simulink subsystem "PvtSubSys_PLAN_AP"  (R2020b)
settings: Solver=VariableStepAuto  StartTime=0.0  StopTime=10.0  RelTol=1e-3
undefined symbols (not defined in the file or in its folder): C_LongCtrl_0_Single, C_LongCtrl_0_Uint8, C_LongCtrl_Mph2Kph, magnitude, P_LongCtrl_accelTargAbsThrd, P_LongCtrl_AddVelAccelChange, P_LongCtrl_AddVelAccelThrd, P_LongCtrl_AddVelDistDesThrd, P_LongCtrl_AddVelEnable, P_LongCtrl_AddVelRefMsThrd, P_LongCtrl_ALaLowerChar, P_LongCtrl_ALaUpperCharEco, P_LongCtrl_ALaUpperCharNormal, P_LongCtrl_ALaUpperCharSport, P_LongCtrl_ALCAccLimitByDangerXAxis, P_LongCtrl_ALCAccLimitByDangerYAxis, P_LongCtrl_ALvAcceleLowerChar, P_LongCtrl_ALvAcceleUpperCharEco, P_LongCtrl_ALvAcceleUpperCharNormal, P_LongCtrl_ALvAcceleUpperCharSport, P_LongCtrl_CCaccelCCNeg2PosJerk, P_LongCtrl_CCaccelCCPosJerk, P_LongCtrl_CCaccelLowerIsLaneChange, P_LongCtrl_CCaccelMaxLCActive, P_LongCtrl_CCaccelMinECOAL, P_LongCtrl_CCaccelMinFastDecel, P_LongCtrl_CCaccelMinNoFastDecel, P_LongCtrl_CCaccelMinNormAL, P_LongCtrl_CCaccelMinSportAL, P_LongCtrl_CCaccelUpperCC, P_LongCtrl_CCaccelUpperCCSafeStop, P_LongCtrl_CCaMinNegAcceleLowerBand, P_LongCtrl_CCaMinNegAcceleUpperBand, P_LongCtrl_CCaMinPosAcceleLowerBand, P_LongCtrl_CCaMinPosAcceleUpperBand, P_LongCtrl_CCbECO, P_LongCtrl_CCbNorm, P_LongCtrl_CCbSport, P_LongCtrl_CCcoefESPSpd2IPSpd1, P_LongCtrl_CCcoefESPSpd2IPSpd2, P_LongCtrl_CCdecelCCJerk, P_LongCtrl_CCdecelCCJerkNegVLCInternalAcc, P_LongCtrl_CCfacNegAcceleLowerBand, P_LongCtrl_CCfacNegAcceleUpperBand, P_LongCtrl_CCfacPosAcceleLowerBand, P_LongCtrl_CCfacPosAcceleUpperBand, P_LongCtrl_CCkECO, P_LongCtrl_CCkNorm, P_LongCtrl_CCkSport, P_LongCtrl_CCLCIncSetSpdAdd, P_LongCtrl_CCLCIncSetSpdAddCntStartValue, P_LongCtrl_CCResumeDelayDeltaVel, P_LongCtrl_CCtAcceleTimeNeg, P_LongCtrl_CCtAcceleTimeNegCorrXAxis, P_LongCtrl_CCtAcceleTimeNegCorrYAxis, P_LongCtrl_CCtAcceleTimePos, P_LongCtrl_CCtAcceleTimePosCorrXAxis, P_LongCtrl_CCtAcceleTimePosCorrYAxis, P_LongCtrl_CCtStepVelPlan, P_LongCtrl_CCtTotVelPlan ... (+150)
libraries: simulink x62, TrueDurationTime x1
(part 5 of 7)

== system PvtSubSys_PLAN_AP/AP/AP/IC/CurvatureOfMapCalc/Chart/velSubjLimChar ==
  LongCtrl_IC_EHRV2_CurMatrixLP : Inport  OutDataTypeStr=single  PortDimensions=[1 10]
  f : TriggerPort  TriggerType=function-call  VariantControl=(inherit)
      settings: CopyFcn=Stateflow.SLINSF.SimulinkMan.removeBlockPreDeleteFcn  PreDeleteFcn=Stateflow.SLINSF.SimulinkMan.unsafePredeleteFcn
  1-D Lookup Table2 : Lookup_n-D  NumberOfTableDimensions=1  BreakpointsForDimension1=P_LongCtrl_ICCurvatureMapLimitSpdXAxis  Table=P_LongCtrl_ICCurvatureMapLimitSpdYAxis  ExtrapMethod=Clip  InternalRulePriority=Speed  RndMeth=Simplest  InputSameDT=on
  Gain2 : Gain  Gain=1/3.6
  velSubjLimMap : Outport
  wires:
  LongCtrl_IC_EHRV2_CurMatrixLP/1 -> 1-D Lookup Table2/1
  1-D Lookup Table2/1 -> Gain2/1
  Gain2/1 -> velSubjLimMap/1

== system PvtSubSys_PLAN_AP/AP/AP/IC/CurvatureOfMapCalc/LP ==
  LongCtrl_IC_EHRV2_CurMatrix : Inport  OutDataTypeStr=single  Partition=on  PartitionDimension=1  PartitionWidth=1  PartitionOffset=0
  Abs : Abs
  Abs1 : Abs
  Add : Sum  Inputs=--+  OutDataTypeStr=single
  Add5 : Sum  Inputs=+-
  Add6 : Sum
  Compare To Constant : simulink/Logic and Bit Operations/Compare To Constant  relop=>=  const=0.15  OutDataTypeStr=boolean
  Constant : Constant  Value=0  OutDataTypeStr=single
  Constant1 : Constant  Value=0.1  OutDataTypeStr=single
  Constant12 : Constant  Value=0.02  OutDataTypeStr=single
  For Each : ForEach  DisableCoverage=on
  Max : MinMax  Function=max
  Min : MinMax
  Product7 : Product  Inputs=*/
  Product8 : Product
  Sum of Elements2 : Sum  Inputs=+
  Switch : Switch  Criteria=u2 > Threshold
  Tapped Delay2 : simulink/Discrete/Tapped Delay  vinit=0.0  samptime=-1  NumDelays=3  DelayOrder=Oldest  includeCurrent=off
  Unit Delay : UnitDelay  SampleTime=-1  HasFrameUpgradeWarning=on
  LongCtrl_IC_EHRV2_CurMatrixLP : Outport  ConcatenationDimension=1
  wires:
  Unit Delay/1 -> Add6/2, Add5/2
  Constant1/1 -> Product7/2
  Min/1 -> Add/2
  Max/1 -> Add/1
  Sum of Elements2/1 -> Add/3
  Constant12/1 -> Product7/1
  Product7/1 -> Product8/1
  Add/1 -> Add5/1
  Add5/1 -> Product8/2
  Product8/1 -> Add6/1
  Add6/1 -> Switch/3
  Tapped Delay2/1 -> Sum of Elements2/1, Max/1, Min/1
  Abs/1 -> LongCtrl_IC_EHRV2_CurMatrixLP/1
  Abs1/1 -> Compare To Constant/1
  Compare To Constant/1 -> Switch/2
  LongCtrl_IC_EHRV2_CurMatrix/1 -> Abs1/1, Tapped Delay2/1
  Switch/1 -> Unit Delay/1, Abs/1
  Constant/1 -> Switch/1

== system PvtSubSys_PLAN_AP/AP/AP/IC/CurvatureOfRoadCalc/If Action Subsystem ==
  L1dC2V : Inport
  L1dC3V : Inport  Port=2
  R1dC2V : Inport  Port=3
  R1dC3V : Inport  Port=4
  L1dDisFront : Inport  Port=5
  R1dDisFront : Inport  Port=6
  L1bIsLineExist : Inport  Port=7
  R1bIsLineExis : Inport  Port=8
  velSubj : Inport  Port=9
  LongCtrl_Line_std : Inport  Port=10
  Action Port : ActionPort
  Abs : Abs
  Constant : Constant  Value=0  OutDataTypeStr=single
  Constant1 : Constant  Value=0  OutDataTypeStr=single
  CurvatureMix : Subsystem
  For Each Subsystem : Subsystem  TreatAsAtomicUnit=on
  Vector Concatenate : Concatenate
  Vector Concatenate1 : Concatenate
  Curvature : Outport
  wires:
  Vector Concatenate1/1 -> For Each Subsystem/4(R1dC3V)
  Constant1/1 -> Vector Concatenate1/1
  Constant/1 -> Vector Concatenate/1
  Vector Concatenate/1 -> For Each Subsystem/2(L1dC3V)
  Abs/1 -> CurvatureMix/1(In1)
  CurvatureMix/1(Out1) -> Curvature/1
  For Each Subsystem/1(Curvature) -> Abs/1  "Curvature"
  velSubj/1 -> For Each Subsystem/9(velSubj)  "velSubj"
  L1dC2V/1 -> For Each Subsystem/1(L1dC2V)
  R1dC2V/1 -> For Each Subsystem/3(R1dC2V)
  L1bIsLineExist/1 -> For Each Subsystem/7(L1bIsLineExist)
  R1bIsLineExis/1 -> For Each Subsystem/8(R1bIsLineExis)
  L1dC3V/1 -> Vector Concatenate/2
  L1dDisFront/1 -> For Each Subsystem/5(L1dDisFront)
  R1dDisFront/1 -> For Each Subsystem/6(R1dDisFront)
  R1dC3V/1 -> Vector Concatenate1/2
  LongCtrl_Line_std/1 -> CurvatureMix/2(LongCtrl_Line_std)

== system PvtSubSys_PLAN_AP/AP/AP/IC/CurvatureOfRoadCalc/If Action Subsystem1 ==
  Action Port : ActionPort
  Constant17 : Constant  Value=0  OutDataTypeStr=single
  Curvature : Outport
  wires:
  Constant17/1 -> Curvature/1

== system PvtSubSys_PLAN_AP/AP/AP/IC/CurvatureOfRoadCalc/LP2 ==
  In1 : Inport
  Add5 : Sum  Inputs=+-
  Add6 : Sum
  Constant12 : Constant  Value=0.02  OutDataTypeStr=single
  Constant13 : Constant  Value=0.3  OutDataTypeStr=single
  Product7 : Product  Inputs=*/
  Product8 : Product
  Unit Delay : UnitDelay  SampleTime=-1  HasFrameUpgradeWarning=on
  Out1 : Outport
  wires:
  Constant12/1 -> Product7/1
  Constant13/1 -> Product7/2
  Product7/1 -> Product8/1
  In1/1 -> Add5/1
  Product8/1 -> Add6/1
  Add6/1 -> Out1/1, Unit Delay/1
  Unit Delay/1 -> Add5/2, Add6/2
  Add5/1 -> Product8/2

== system PvtSubSys_PLAN_AP/AP/AP/IC/Subsystem1/Subsystem ==
  In1 : Inport
  Add : Sum  Inputs=--+  OutDataTypeStr=single
  Add1 : Sum  Inputs=--+  OutDataTypeStr=single
  Demux : Demux  Outputs=2
  Max : MinMax  Function=max
  Max1 : MinMax  Function=max
  Min : MinMax
  Min1 : MinMax
  Mux : Mux  Inputs=2
  Sum of Elements1 : Sum  Inputs=+
  Sum of Elements2 : Sum  Inputs=+
  Tapped Delay1 : simulink/Discrete/Tapped Delay  vinit=0.0  samptime=-1  NumDelays=3  DelayOrder=Oldest  includeCurrent=off
  Tapped Delay2 : simulink/Discrete/Tapped Delay  vinit=0.0  samptime=-1  NumDelays=3  DelayOrder=Oldest  includeCurrent=off
  Line_stdK1 : Outport
  wires:
  Tapped Delay2/1 -> Max/1, Min/1, Sum of Elements2/1
  Max/1 -> Add/1
  Min/1 -> Add/2
  Sum of Elements2/1 -> Add/3
  In1/1 -> Demux/1
  Sum of Elements1/1 -> Add1/3
  Min1/1 -> Add1/2
  Max1/1 -> Add1/1
  Tapped Delay1/1 -> Sum of Elements1/1, Min1/1, Max1/1
  Demux/1 -> Tapped Delay1/1
  Demux/2 -> Tapped Delay2/1
  Add1/1 -> Mux/1
  Add/1 -> Mux/2
  Mux/1 -> Line_stdK1/1

== system PvtSubSys_PLAN_AP/AP/AP/IC/Subsystem1/Subsystem1 ==
  In1 : Inport
  Demux4 : Demux  Outputs=2
  Gain : Gain  Gain=0.04  OutDataTypeStr=single
  Gain1 : Gain  Gain=0.04  ParamDataTypeStr=single
  Mux1 : Mux  Inputs=2
  Sum of Elements : Sum  Inputs=+
  Sum of Elements1 : Sum  Inputs=+
  Tapped Delay : simulink/Discrete/Tapped Delay  vinit=0.0  samptime=-1  NumDelays=25  DelayOrder=Oldest  includeCurrent=off
  Tapped Delay1 : simulink/Discrete/Tapped Delay  vinit=0.0  samptime=-1  NumDelays=25  DelayOrder=Oldest  includeCurrent=off
  Out1 : Outport
  wires:
  Sum of Elements1/1 -> Gain1/1
  Mux1/1 -> Out1/1
  Gain1/1 -> Mux1/2
  Tapped Delay/1 -> Sum of Elements/1
  Demux4/1 -> Tapped Delay/1
  Sum of Elements/1 -> Gain/1
  Gain/1 -> Mux1/1
  Tapped Delay1/1 -> Sum of Elements1/1
  Demux4/2 -> Tapped Delay1/1
  In1/1 -> Demux4/1

== system PvtSubSys_PLAN_AP/AP/AP/SJ/DeceleToStop/DeceleToStop/DresCalc ==
  distTargRel : Inport  OutDataTypeStr=single  PortDimensions=1
  f : TriggerPort  TriggerType=function-call  VariantControl=Variant
      settings: CopyFcn=Stateflow.SLINSF.SimulinkMan.removeBlockPreDeleteFcn  PreDeleteFcn=Stateflow.SLINSF.SimulinkMan.unsafePredeleteFcn
  Add : Sum  Inputs=+-
  P_LongCtrl_SJdStop : Constant  Value=P_LongCtrl_SJdStop
  distRes : Outport
  wires:
  P_LongCtrl_SJdStop/1 -> Add/2
  Add/1 -> distRes/1  "distRes"
  distTargRel/1 -> Add/1  "distTargRel"

== system PvtSubSys_PLAN_AP/AP/AP/SJ/DeceleToStop/DeceleToStop/VxTargetCalc ==
  velSubj : Inport  OutDataTypeStr=single  PortDimensions=1
  velTargetRel : Inport  Port=2  OutDataTypeStr=single  PortDimensions=1
  f : TriggerPort  TriggerType=function-call  VariantControl=Variant
      settings: CopyFcn=Stateflow.SLINSF.SimulinkMan.removeBlockPreDeleteFcn  PreDeleteFcn=Stateflow.SLINSF.SimulinkMan.unsafePredeleteFcn
  Add : Sum
  velTargetAbs : Outport
  wires:
  Add/1 -> velTargetAbs/1  "velTargetAbs"
  velSubj/1 -> Add/1  "velSubj"
  velTargetRel/1 -> Add/2  "velTargetRel"

== system PvtSubSys_PLAN_AP/AP/AP/SJ/DisBar/ACC_DisplayBar1 ==
  TimeGap : Inport
  DesireDistance : Inport  Port=2
  ACCmode : Inport  Port=3
  TargetRange : Inport  Port=4  Partition=on  PartitionDimension=1  PartitionWidth=1  PartitionOffset=0
  Scale : Inport  Port=5
  TargetExist : Inport  Port=6  Partition=on  PartitionDimension=1  PartitionWidth=1  PartitionOffset=0
  ACC_DisplayBar : MATLAB Function  TreatAsAtomicUnit=on
  For Each : ForEach  DisableCoverage=on
  Unit Delay34 : UnitDelay  SampleTime=-1  HasFrameUpgradeWarning=on
  Signal_ACC_TgtObjBarDisp : Outport  ConcatenationDimension=1
  wires:
  TargetExist/1 -> ACC_DisplayBar/6(TargetExist)  "TargetExist"
  Scale/1 -> ACC_DisplayBar/5(Scale)  "Scale"
  TargetRange/1 -> ACC_DisplayBar/4(TargetRange)  "TargetRange"
  ACCmode/1 -> ACC_DisplayBar/3(ACCmode)  "ACCmode"
  DesireDistance/1 -> ACC_DisplayBar/2(DesireDistance)  "DesireDistance"
  TimeGap/1 -> ACC_DisplayBar/1(TimeGap)  "TimeGap"
  Unit Delay34/1 -> ACC_DisplayBar/7(DisplayBarK1)
  ACC_DisplayBar/1(DisplayBar) -> Unit Delay34/1, Signal_ACC_TgtObjBarDisp/1  "Signal_ACC_TgtObjBarDisp"

== system PvtSubSys_PLAN_AP/AP/AP/SJ/TakeOver/Gap ==
  distTargetRel : Inport
  velSubj : Inport  Port=2
  Constant : Constant  Value=0.1  OutDataTypeStr=single
  MinMax : MinMax  Function=max  Inputs=2
  Product : Product  Inputs=*/
  gap : Outport
  wires:
  MinMax/1 -> Product/2
  Constant/1 -> MinMax/2
  Product/1 -> gap/1
  velSubj/1 -> MinMax/1
  distTargetRel/1 -> Product/1

== system PvtSubSys_PLAN_AP/AP/AP/FollowCtrl/DecelToStopCtrl/DecelToStopCtrl/P_LongCtrl_velSubjThresEnableStopAdd ==
  distTargRel : Inport
  velSubjThresForceStop : Inport  Port=2
  1-D Lookup Table : Lookup_n-D  NumberOfTableDimensions=1  BreakpointsForDimension1=P_LongCtrl_FollowvelSubjThresEnableStopAddXAxis  Table=P_LongCtrl_FollowvelSubjThresEnableStopAddYAxis  ExtrapMethod=Clip  InternalRulePriority=Speed  RndMeth=Simplest  InputSameDT=on
  1-D Lookup Table1 : Lookup_n-D  NumberOfTableDimensions=1  BreakpointsForDimension1=P_LongCtrl_FollowaccelFollowDesThresEnableStopXAxis  Table=P_LongCtrl_FollowaccelFollowDesThresEnableStopYAxis  ExtrapMethod=Clip  InternalRulePriority=Speed  RndMeth=Simplest  InputSameDT=on
  Add : Sum  Inputs=+-
  Add1 : Sum
  Constant : Constant  Value=P_LongCtrl_FollowDistDiff2VelSubjThresEnableStop
  Lookup Table Dynamic : simulink/Lookup Tables/Lookup Table Dynamic  LookUpMeth=Interpolation-Use End Values  OutDataType=fixdt('single')  OutScaling=[]  OutputDataTypeScalingMode=Specify via dialog  OutDataTypeStr=single  DoSatur=off
  P_LongCtrl_FollowdistDesStopMin : Constant  Value=P_LongCtrl_FollowdistDesStopMin  OutDataTypeStr=single
  P_LongCtrl_FollowvelSubjThresEnableStop : Constant  Value=P_LongCtrl_FollowvelSubjThresEnableStop  OutDataTypeStr=single
  P_LongCtrl_FollowvelSubjThresEnableStop1 : Constant  Value=P_LongCtrl_FollowVelSubjForceStopEnable  OutDataTypeStr=single
  Switch : Switch  Criteria=u2 > Threshold
  Vector Concatenate : Concatenate
  accelFollowDesThresEnableStop : Outport
  velSubjThresEnableStopAdd : Outport  Port=2
  velSubjThresForceStopStationaryTarget : Outport  Port=3
  wires:
  distTargRel/1 -> 1-D Lookup Table1/1, Add/2
  P_LongCtrl_FollowdistDesStopMin/1 -> Add/1
  Add/1 -> Lookup Table Dynamic/1, 1-D Lookup Table/1
  1-D Lookup Table/1 -> Add1/2, velSubjThresEnableStopAdd/1  "LongCtrl_velSubjThresEnableStopAdd"
  1-D Lookup Table1/1 -> accelFollowDesThresEnableStop/1  "LongCtrl_accelFollowDesThresEnableStop"
  Constant/1 -> Lookup Table Dynamic/2
  velSubjThresForceStop/1 -> Vector Concatenate/1
  Add1/1 -> Switch/3, Vector Concatenate/2
  Vector Concatenate/1 -> Lookup Table Dynamic/3
  Switch/1 -> velSubjThresForceStopStationaryTarget/1  "LongCtrl_velSubjThresForceStopStationaryTarget"
  P_LongCtrl_FollowvelSubjThresEnableStop/1 -> Add1/1
  P_LongCtrl_FollowvelSubjThresEnableStop1/1 -> Switch/2
  Lookup Table Dynamic/1 -> Switch/1

== system PvtSubSys_PLAN_AP/AP/AP/FollowCtrl/DecelToStopCtrl/DecelToStopCtrl/Subsystem ==
  axvRoadSlopeMs2 : Inport
  P_LongCtrl_FollowaccelForceStopMinChar : Lookup_n-D  NumberOfTableDimensions=1  BreakpointsForDimension1=P_LongCtrl_FollowaccelForceStopMinCharXAxis  Table=P_LongCtrl_FollowaccelForceStopMinCharYAxis  ExtrapMethod=Clip  InternalRulePriority=Speed  OutDataTypeStr=single  RndMeth=Simplest  InputSameDT=on
  P_LongCtrl_jerkForceStopChar : Lookup_n-D  NumberOfTableDimensions=1  BreakpointsForDimension1=P_LongCtrl_FollowjerkForceStopCharXAxis  Table=P_LongCtrl_FollowjerkForceStopCharYAxis  ExtrapMethod=Clip  InternalRulePriority=Speed  RndMeth=Simplest  InputSameDT=on
  P_LongCtrl_velSubjThresForceStopChar : Lookup_n-D  NumberOfTableDimensions=1  BreakpointsForDimension1=P_LongCtrl_FollowVelSubjThresForceStopXAxis  Table=P_LongCtrl_FollowVelSubjThresForceStopYAxis  ExtrapMethod=Clip  InternalRulePriority=Speed  RndMeth=Simplest  InputSameDT=on
  velSubjThresForceStop : Outport
  jerkForceStop : Outport  Port=2
  accelForceMin : Outport  Port=3
  wires:
  axvRoadSlopeMs2/1 -> P_LongCtrl_FollowaccelForceStopMinChar/1, P_LongCtrl_jerkForceStopChar/1, P_LongCtrl_velSubjThresForceStopChar/1
  P_LongCtrl_velSubjThresForceStopChar/1 -> velSubjThresForceStop/1  "LongCtrl_velSubjThresForceStop"
  P_LongCtrl_jerkForceStopChar/1 -> jerkForceStop/1  "LongCtrl_jerkForceStop"
  P_LongCtrl_FollowaccelForceStopMinChar/1 -> accelForceMin/1  "LongCtrl_accelForceMin"

== system PvtSubSys_PLAN_AP/AP/AP/FollowCtrl/FollowBandJerkCalc/DecelFollowJerkCalc/OverrideJerk/lowerJerkOverrideCalc ==
  VlcInternalAccK1 : Inport  OutDataTypeStr=single  PortDimensions=1
  f : TriggerPort  TriggerType=function-call  VariantControl=Variant
      settings: CopyFcn=Stateflow.SLINSF.SimulinkMan.removeBlockPreDeleteFcn  PreDeleteFcn=Stateflow.SLINSF.SimulinkMan.unsafePredeleteFcn
  1-D Lookup Table : Lookup_n-D  NumberOfTableDimensions=1  BreakpointsForDimension1=[0 1 2 3]  Table=[-4 -10 -20 -30]  ExtrapMethod=Clip  InternalRulePriority=Speed  RndMeth=Simplest  InputSameDT=on
  lowerJerkOverride : Outport
  wires:
  1-D Lookup Table/1 -> lowerJerkOverride/1
  VlcInternalAccK1/1 -> 1-D Lookup Table/1

== system PvtSubSys_PLAN_AP/AP/AP/IC/CurvatureOfRoadCalc/If Action Subsystem/CurvatureMix ==
  In1 : Inport
  LongCtrl_Line_std : Inport  Port=2
  2-D Lookup Table1 : Lookup_n-D  BreakpointsForDimension1=P_LongCtrl_ICcoefCurvatureCharX1  BreakpointsForDimension2=P_LongCtrl_ICcoefCurvatureCharX2  Table=P_LongCtrl_ICcoefCurvatureCharY  ExtrapMethod=Clip  InternalRulePriority=Speed  RndMeth=Simplest  InputSameDT=on
      settings: InputPortMap=u0,u1
  Add : Sum  Inputs=+-
  Add1 : Sum
  Constant : Constant  OutDataTypeStr=single
  Demux : Demux  Outputs=2
  LP : Subsystem
  Product : Product
  Product1 : Product
  Signal Conversion : SignalConversion  OverrideOpt=off
  Signal Conversion1 : SignalConversion  OverrideOpt=off
  Out1 : Outport
  wires:
  Signal Conversion1/1 -> Product1/2, 2-D Lookup Table1/2  "LongCtrl_curvatureWithC3"
  Signal Conversion/1 -> Product/1, 2-D Lookup Table1/1  "LongCtrl_curvatureNoC3"
  Demux/1 -> Signal Conversion/1
  Add1/1 -> LP/1(In1)  "LongCtrl_curvatureForCurveDecelRaw"
  Demux/2 -> Signal Conversion1/1
  In1/1 -> Demux/1
  2-D Lookup Table1/1 -> Product/2, Add/2  "LongCtrl_coefCurvatureNoC3"
  Product1/1 -> Add1/2
  Product/1 -> Add1/1
  Add/1 -> Product1/1  "LongCtrl_coefCurvatureWithC3"
  Constant/1 -> Add/1
  LP/1(Out1) -> Out1/1
  LongCtrl_Line_std/1 -> LP/2(LongCtrl_Line_std)

== system PvtSubSys_PLAN_AP/AP/AP/IC/CurvatureOfRoadCalc/If Action Subsystem/For Each Subsystem ==
  L1dC2V : Inport
  L1dC3V : Inport  Port=2  Partition=on  PartitionDimension=1  PartitionWidth=1  PartitionOffset=0
  R1dC2V : Inport  Port=3
  R1dC3V : Inport  Port=4  Partition=on  PartitionDimension=1  PartitionWidth=1  PartitionOffset=0
  L1dDisFront : Inport  Port=5
  R1dDisFront : Inport  Port=6
  L1bIsLineExist : Inport  Port=7
  R1bIsLineExis : Inport  Port=8
  velSubj : Inport  Port=9
  CurvatureChar : Stateflow chart  TreatAsAtomicUnit=on
  For Each : ForEach  DisableCoverage=on
  Curvature : Outport  ConcatenationDimension=1
  wires:
  CurvatureChar/1(CurvatureIFC) -> Curvature/1  "Curvature"
  R1dC3V/1 -> CurvatureChar/7(GetR1dC3V)
  R1bIsLineExis/1 -> CurvatureChar/2(R1bIsLineExis)
  L1dDisFront/1 -> CurvatureChar/5(GetL1dDisFront)
  L1dC3V/1 -> CurvatureChar/4(GetL1dC3V)
  L1bIsLineExist/1 -> CurvatureChar/1(L1bIsLineExist)
  L1dC2V/1 -> CurvatureChar/3(GetL1dC2V)
  R1dC2V/1 -> CurvatureChar/6(GetR1dC2V)
  R1dDisFront/1 -> CurvatureChar/8(GetR1dDisFront)
  velSubj/1 -> CurvatureChar/9(velSubj)  "velSubj"

== system PvtSubSys_PLAN_AP/AP/AP/IC/CurvatureOfRoadCalc/If Action Subsystem/CurvatureMix/LP ==
  In1 : Inport
  LongCtrl_Line_std : Inport  Port=2
  1-D Lookup Table : Lookup_n-D  NumberOfTableDimensions=1  BreakpointsForDimension1=[0 0.3 0.6 0.9 1.2 1.5]  Table=[0.3 0.3 0.6 0.9 1.2 1.5]  InternalRulePriority=Speed  RndMeth=Simplest  InputSameDT=on
  Add : Sum  Inputs=--+  OutDataTypeStr=single
  Add5 : Sum  Inputs=+-
  Add6 : Sum
  Constant12 : Constant  Value=0.02  OutDataTypeStr=single
  Max : MinMax  Function=max
  Min : MinMax
  Product7 : Product  Inputs=*/
  Product8 : Product
  Sum of Elements2 : Sum  Inputs=+
  Tapped Delay2 : simulink/Discrete/Tapped Delay  vinit=0.0  samptime=-1  NumDelays=3  DelayOrder=Oldest  includeCurrent=off
  Unit Delay : UnitDelay  SampleTime=-1  HasFrameUpgradeWarning=on
  Out1 : Outport
  wires:
  Add5/1 -> Product8/2
  Unit Delay/1 -> Add6/2, Add5/2
  Add6/1 -> Unit Delay/1, Out1/1
  Product8/1 -> Add6/1
  Add/1 -> Add5/1
  Product7/1 -> Product8/1
  Constant12/1 -> Product7/1
  Tapped Delay2/1 -> Sum of Elements2/1, Max/1, Min/1
  Sum of Elements2/1 -> Add/3
  Max/1 -> Add/1
  Min/1 -> Add/2
  In1/1 -> Tapped Delay2/1
  1-D Lookup Table/1 -> Product7/2
  LongCtrl_Line_std/1 -> 1-D Lookup Table/1

== system PvtSubSys_PLAN_AP/AP/AP/IC/CurvatureOfRoadCalc/If Action Subsystem/For Each Subsystem/CurvatureChar/Curvature1Calc ==
  note: Curature=6*C3*X+2*C2;
      | Curature=(CuratureL+CuratureR)/2
  GetL1dC2V : Inport
  GetL1dC3V : Inport  Port=2
  GetR1dC2V : Inport  Port=3
  GetR1dC3V : Inport  Port=4
  GetL1dDisFront : Inport  Port=5
  GetR1dDisFront : Inport  Port=6
  velSubj : Inport  Port=7
  f : TriggerPort  TriggerType=function-call  VariantControl=Variant
      settings: CopyFcn=Stateflow.SLINSF.SimulinkMan.removeBlockPreDeleteFcn  PreDeleteFcn=Stateflow.SLINSF.SimulinkMan.unsafePredeleteFcn
  1-D Lookup Table1 : Lookup_n-D  NumberOfTableDimensions=1  BreakpointsForDimension1=[11.1 27.7]  Table=[35 90]  ExtrapMethod=Clip  InternalRulePriority=Speed  RndMeth=Simplest  InputSameDT=on
  Add1 : Sum
  Add3 : Sum
  Add4 : Sum
  Constant1 : Constant  Value=2  OutDataTypeStr=single
  Constant11 : Constant  Value=0.5  OutDataTypeStr=single
  Constant2 : Constant  Value=6  OutDataTypeStr=single
  Constant8 : Constant  Value=2  OutDataTypeStr=single
  Constant9 : Constant  Value=6  OutDataTypeStr=single
  MinMax : MinMax  Inputs=2
  MinMax1 : MinMax  Inputs=2
  Product{,1..6} (7 alike) : Product
  Curvature1 : Outport
  wires:
  Product6/1 -> Curvature1/1
  1-D Lookup Table1/1 -> MinMax/2, MinMax1/1
  velSubj/1 -> 1-D Lookup Table1/1
  GetL1dDisFront/1 -> MinMax/1
  Constant1/1 -> Product/2
  Add3/1 -> Add4/2
  GetR1dC2V/1 -> Product3/1
  Product1/1 -> Product2/1
  Product5/1 -> Add3/2
  GetR1dDisFront/1 -> MinMax1/2
  Product3/1 -> Add3/1
  Constant2/1 -> Product1/2
  GetL1dC2V/1 -> Product/1
  Product2/1 -> Add1/2
  MinMax1/1 -> Product5/2
  Constant8/1 -> Product3/2
  MinMax/1 -> Product2/2
  Product4/1 -> Product5/1
  Constant11/1 -> Product6/2
  Add4/1 -> Product6/1
  GetL1dC3V/1 -> Product1/1
  GetR1dC3V/1 -> Product4/1
  Add1/1 -> Add4/1
  Product/1 -> Add1/1
  Constant9/1 -> Product4/2

== system PvtSubSys_PLAN_AP/AP/AP/IC/CurvatureOfRoadCalc/If Action Subsystem/For Each Subsystem/CurvatureChar/Curvature2Calc ==
  note: Curature=6*C3*X+2*C2;
  GetL1dC2V : Inport
  GetL1dC3V : Inport  Port=2
  GetL1dDisFront : Inport  Port=3
  velSubj : Inport  Port=4
  f : TriggerPort  TriggerType=function-call  VariantControl=Variant
      settings: CopyFcn=Stateflow.SLINSF.SimulinkMan.removeBlockPreDeleteFcn  PreDeleteFcn=Stateflow.SLINSF.SimulinkMan.unsafePredeleteFcn
  1-D Lookup Table2 : Lookup_n-D  NumberOfTableDimensions=1  BreakpointsForDimension1=[11.1 27.7]  Table=[35 90]  ExtrapMethod=Clip  InternalRulePriority=Speed  RndMeth=Simplest  InputSameDT=on
  Add1 : Sum
  Constant1 : Constant  Value=2  OutDataTypeStr=single
  Constant2 : Constant  Value=6  OutDataTypeStr=single
  MinMax : MinMax  Inputs=2
  Product : Product
  Product1 : Product
  Product2 : Product
  Curvature2 : Outport
  wires:
  1-D Lookup Table2/1 -> MinMax/2
  velSubj/1 -> 1-D Lookup Table2/1
  Product2/1 -> Add1/2
  Constant2/1 -> Product1/2
  GetL1dC2V/1 -> Product/1
  GetL1dDisFront/1 -> MinMax/1
  Constant1/1 -> Product/2
  MinMax/1 -> Product2/2
  Product1/1 -> Product2/1
  Add1/1 -> Curvature2/1
  GetL1dC3V/1 -> Product1/1
  Product/1 -> Add1/1

== system PvtSubSys_PLAN_AP/AP/AP/IC/CurvatureOfRoadCalc/If Action Subsystem/For Each Subsystem/CurvatureChar/Curvature3Calc ==
  note: Curature=6*C3*X+2*C2;
  GetR1dC2V : Inport
  GetR1dC3V : Inport  Port=2
  GetR1dDisFront : Inport  Port=3
  velSubj : Inport  Port=4
  f : TriggerPort  TriggerType=function-call  VariantControl=Variant
      settings: CopyFcn=Stateflow.SLINSF.SimulinkMan.removeBlockPreDeleteFcn  PreDeleteFcn=Stateflow.SLINSF.SimulinkMan.unsafePredeleteFcn
  1-D Lookup Table2 : Lookup_n-D  NumberOfTableDimensions=1  BreakpointsForDimension1=[11.1 27.7]  Table=[35 90]  ExtrapMethod=Clip  InternalRulePriority=Speed  RndMeth=Simplest  InputSameDT=on
  Add3 : Sum
  Constant8 : Constant  Value=2  OutDataTypeStr=single
  Constant9 : Constant  Value=6  OutDataTypeStr=single
  MinMax : MinMax  Inputs=2
  Product3 : Product
  Product4 : Product
  Product5 : Product
  Curvature3 : Outport
  wires:
  1-D Lookup Table2/1 -> MinMax/2
  velSubj/1 -> 1-D Lookup Table2/1
  GetR1dC2V/1 -> Product3/1
  Product5/1 -> Add3/2
  GetR1dDisFront/1 -> MinMax/1
  Product3/1 -> Add3/1
  Add3/1 -> Curvature3/1
  MinMax/1 -> Product5/2
  Constant8/1 -> Product3/2
  Product4/1 -> Product5/1
  GetR1dC3V/1 -> Product4/1
  Constant9/1 -> Product4/2

== matlab function PvtSubSys_PLAN_AP/AP/AP/FollowCtrl/VelPlan/AccelCorr ==
  data: num input single; distTargRel input single; distDesCur input single; velRelPlan input single; accelSubjPlan input single; coefAccelCorr output single
function coefAccelCorr = fcn(num,distTargRel,distDesCur,velRelPlan,accelSubjPlan)
velRelPlanOpt=single(zeros(1,40));
velRelPlanOpt(1,:)=velRelPlan(num,:);
velRelPlanMin=single(0);
if (distTargRel>distDesCur)&&(accelSubjPlan>0.2)
   for j=1:40
       if j==1
           velRelPlanMin=velRelPlanOpt(1,1);
       end
       if velRelPlan(j)<velRelPlanMin
           velRelPlanMin=velRelPlan(j);
       end
   end
   coefAccelCorr=intrepolate(single(-5),single(0.95),single(-0.5),single(1),velRelPlanMin);  
else
   coefAccelCorr=single(1); 
end

function result=intrepolate(x1,y1,x2,y2,x)
if x<x1
    result=single(y1);
else
    if x>x2
        result=single(y2);
    else
        result=single(y1+(y2-y1)/(x2-x1)*(x-x1));
    end
end

== matlab function PvtSubSys_PLAN_AP/AP/AP/FollowCtrl/VelPlan/CoefCalc ==
  data: velSubj input single; distTargRel input single; velTargRel input single; distDesCur input single; coefDistEnlarge output single; accelTargAbsFilt input single; coefVelEnlarge output single; P_LongCtrl_FollowcoefDistEnlargeDecToStop parameter single; P_LongCtrl_FollowcoefVelEnlargeDecToStop parameter single
function [coefDistEnlarge,coefVelEnlarge]= CoefCompensionCalc(velSubj,distTargRel,velTargRel,distDesCur,accelTargAbsFilt,P_LongCtrl_FollowcoefDistEnlargeDecToStop,P_LongCtrl_FollowcoefVelEnlargeDecToStop)
distDesCurCoef=distDesCur*single(0.9);
coefIni=single(1);
%% start up or decelerate to stop
if ((velTargRel<-0.2)&&(distTargRel<distDesCurCoef)&&(velSubj<5))
    coefDistEnlarge=P_LongCtrl_FollowcoefDistEnlargeDecToStop;
    coefVelEnlarge=P_LongCtrl_FollowcoefVelEnlargeDecToStop;
else
    if (distDesCur<distTargRel)&&(velSubj<5)&&(accelTargAbsFilt>0.5)
        coefDistEnlarge=single(intrepolate(single(0),single(5),single(5),single(0),velSubj));
        coefVelEnlarge=single(intrepolate(single(0),single(5),single(5),single(0),velSubj));
    else
        coefDistEnlarge=coefIni;
        coefVelEnlarge=coefIni;
    end
end
timesDistRelVSDes=distTargRel/distDesCur;
if timesDistRelVSDes>1.5&&velSubj>5
    coefTemp=intrepolate(single(5),single(1),single(10),single(0.5),velSubj);
    coefDistEnlarge=intrepolate(single(1.5),single(1),single(2),single(0.3),timesDistRelVSDes);
    coefDistEnlarge=coefDistEnlarge*coefTemp;
    coefVelEnlarge=intrepolate(single(1.5),single(1),single(2),single(0.3),timesDistRelVSDes);
    coefVelEnlarge=coefVelEnlarge*coefTemp;
end
if velTargRel>2&&velSubj>5
   coefTemp=intrepolate(single(1),single(1),single(5),single(0.3),velTargRel); 
   coefDistEnlarge=coefDistEnlarge*coefTemp;
   coefVelEnlarge=coefVelEnlarge*coefTemp;
end
function result=intrepolate(x1,y1,x2,y2,x)
if x<x1
    result=single(y1);
else
    if x>x2
        result=single(y2);
    else
        result=single(y1+(y2-y1)/(x2-x1)*(x-x1));
    end
end

== matlab function PvtSubSys_PLAN_AP/AP/AP/FollowCtrl/VelPlan/spdPlanning ==
  data: distTargPlan input single; tTargStop input single; distDesPlan input single; IDP0 input uint8; a0 input single; Vterminate input single; Dterminate input single; afRaw input single; vf input single; R input single; v0 input single; distRelPlanOpt output single; distRelPlan output single; velRelPlanOpt output single; velRelPlan output single; DesVelSubj output single size=[1 40]; accelSubjPlan output single size=[1 40]; J output single; accelSubjPlanTemp output single; dtAccelSubjPlanTemp output single; C0 output single; C1 output single; C2 output single; C3 output single; C4 output single; C5 output single; velSubjPre output single; JadtA output single; JadtADist output single; asum output single; coefJEnlarge output single; distRelPlanMin output single; distRelDesDistRelPlanNumMin output single; tOverride2Active output single; Wd input single; Wv input single; distDesCur input single; velTargRel input single; distTargRel input single; ttc input single; velSubjNegToleranceAdd input single; ACCModeSts input uint8; tCycle input single; accelSubjPlanK1 input single; tOverride2ActiveK1 input single; num output single; numK1 input single; P_LongCtrl_FollowRateJDirStep parameter single; P_LongCtrl_FollowRateJConditionStep parameter single; P_LongCtrl_FollowVelTargetAbsSmoothNum parameter single
function [distRelPlanOpt,distRelPlan,velRelPlanOpt,velRelPlan,DesVelSubj,accelSubjPlan,J,accelSubjPlanTemp,dtAccelSubjPlanTemp,C0,C1,C2,C3,C4,C5,velSubjPre,JadtA,JadtADist,asum,coefJEnlarge,distRelPlanMin,distRelDesDistRelPlanNumMin,tOverride2Active,num] = fcn(distTargPlan,tTargStop,distDesPlan,IDP0,a0,Vterminate,Dterminate,afRaw,vf,R,v0,Wd,Wv,distDesCur,velTargRel,distTargRel,ttc,velSubjNegToleranceAdd,ACCModeSts,tCycle,accelSubjPlanK1,tOverride2ActiveK1,numK1, P_LongCtrl_FollowRateJDirStep, P_LongCtrl_FollowRateJConditionStep, P_LongCtrl_FollowVelTargetAbsSmoothNum)
 s=single(zeros(20,40));
 distRelPlan=single(zeros(20,40));
 v=single(zeros(20,40));
 velRelPlan=single(zeros(20,40));
 velSubjPre=single(zeros(20,40));
 J=single(zeros(20,1));
 coefJEnlarge=single(zeros(20,1));
 JadtA=single(zeros(20,1));
 JadtADist=single(zeros(20,1));
 asum=single(zeros(20,1));
 adetsum=single(zeros(20,1));
 tsum=single(zeros(20,1));
 dsum=single(zeros(20,1));
 vsum=single(zeros(20,1));
 accelSubjPlanTemp=single(zeros(20,40));
 dtAccelSubjPlanTemp=single(zeros(20,40));
 C0=single(zeros(20,1));
 C1=single(zeros(20,1));
 C2=single(zeros(20,1));
 C3=single(zeros(20,1));
 C4=single(zeros(20,1));
 C5=single(zeros(20,1));
 distDesPlanExpand=single(zeros(40,1));
 vTerminateExpand=single(zeros(40,1));
 jTargStop=fix(single(2)*tTargStop);
 velAllIsNeg=false;
 distRelPlanReasonable=true;
 distRelPlanStartReasonable=true;
 Wa=single(1);
 Wadet=single(1);
 tOverride2Active=tOverride2ActiveK1;
 iStart=single(1);
 iEnd=single(20);
 persistent cntSmallNumRawArb;
 if isempty(cntSmallNumRawArb)
     cntSmallNumRawArb=single(0);
 end
 persistent cntBigNumRawArb;
 if isempty(cntBigNumRawArb)
     cntBigNumRawArb=single(0);
 end
 smallNumArbFail=true;
 BigNumArbFail=true;
 % A42=t;
 A42=single([0.5 1.5 2.5 3.5 4.5 5.5 6.5 7.5 8.5 9.5 10.5 11.5 12.5 13.5 14.5 15.5 16.5 17.5 18.5 19.5]);
 % A43=t^2;
 A43=single([0.25 2.25 6.25 12.25 20.25 30.25 42.25 56.25 72.25 90.25 110.25 132.25 156.25 182.25 210.25 240.25 272.25 306.25 342.25 380.25]);
 % A44=t^3;
 A44=single([0.125 3.375 15.625 42.875 91.125 166.375 274.625 421.875 614.125 857.375 1157.625 1520.875 1953.125 2460.375 3048.625 3723.875 4492.125 5359.375 6331.625 7414.875]);
 % A45=t^4;
 A45=single([0.0625 5.0625 39.0625 150.0625 410.0625 915.0625 1785.0625 3164.0625 5220.0625 8145.0625 12155.0625 17490.0625 24414.0625 33215.0625 44205.0625 57720.0625 74120.0625 93789.0625 117135.0625 144590.0625]);
 % A46=t^5;
 A46=single([0.03125 7.59375 97.65625 525.21875 1845.28125 5032.84375 11602.90625 23730.46875 44370.53125 77378.09375 127628.15625 201135.71875 305175.78125 448403.34375 640973.40625 894660.96875 1222981.03125 1641308.59375 2166998.65625 2819506.21875]);
 %A53=2*t;
 A53=single([1,3,5,7,9,11,13,15,17,19,21,23,25,27,29,31,33,35,37,39]);
 %A54=3*t^2;
 A54=single([0.75,6.75,18.75,36.75,60.75,90.75,126.75,168.75,216.75,270.75,330.75,396.75,468.75,546.75,630.75,720.75,816.75,918.75,1026.75,1140.75]);
 %A55=4*t^3;
 A55=single([0.5,13.5,62.5,171.5,364.5,665.5,1098.5,1687.5,2456.5,3429.5,4630.5,6083.5,7812.5,9841.5,12194.5,14895.5,17968.5,21437.5,25326.5,29659.5]);
 %A56=5*t^4;
 A56=single([0.3125,25.3125,195.3125,750.3125,2050.3125,4575.3125,8925.3125,15820.3125,26100.3125,40725.3125,60775.3125,87450.3125,122070.3125,166075.3125,221025.3125,288600.3125,370600.3125,468945.3125,585675.3125,722950.3125]);
 %A64=6*t;
 A64=single([3,9,15,21,27,33,39,45,51,57,63,69,75,81,87,93,99,105,111,117]);
 %A65=12*t^2;
 A65=single([3,27,75,147,243,363,507,675,867,1083,1323,1587,1875,2187,2523,2883,3267,3675,4107,4563]);
 %A66=20*t^3;
 A66=single([2.5,67.5,312.5,857.5,1822.5,3327.5,5492.5,8437.5,12282.5,17147.5,23152.5,30417.5,39062.5,49207.5,60972.5,74477.5,89842.5,107187.5,126632.5,148297.5]);
 
 %tBack1=(0.5*j)
 tBack1=single([0.5,1,1.5,2,2.5,3,3.5,4,4.5,5,5.5,6,6.5,7,7.5,8,8.5,9,9.5,10,10.5,11,11.5,12,12.5,13,13.5,14,14.5,15,15.5,16,16.5,17,17.5,18,18.5,19,19.5,20]);
 %tBack2=(0.5*j)^2
 tBack2=single([0.25,1,2.25,4,6.25,9,12.25,16,20.25,25,30.25,36,42.25,49,56.25,64,72.25,81,90.25,100,110.25,121,132.25,144,156.25,169,182.25,196,210.25,225,240.25,256,272.25,289,306.25,324,342.25,361,380.25,400]);
 %tBack3=(0.5*j)^3
 tBack3=single([0.125,1,3.375,8,15.625,27,42.875,64,91.125,125,166.375,216,274.625,343,421.875,512,614.125,729,857.375,1000,1157.625,1331,1520.875,1728,1953.125,2197,2460.375,2744,3048.625,3375,3723.875,4096,4492.125,4913,5359.375,5832,6331.625,6859,7414.875,8000]);
 %tBack4=(0.5*j)^4
 tBack4=single([0.0625,1,5.0625,16,39.0625,81,150.0625,256,410.0625,625,915.0625,1296,1785.0625,2401,3164.0625,4096,5220.0625,6561,8145.0625,10000,12155.0625,14641,17490.0625,20736,24414.0625,28561,33215.0625,38416,44205.0625,50625,57720.0625,65536,74120.0625,83521,93789.0625,104976,117135.0625,130321,144590.0625,160000]);
 %tBack5=(0.5*j)^5
 tBack5=single([0.03125,1,7.59375,32,97.65625,243,525.21875,1024,1845.28125,3125,5032.84375,7776,11602.90625,16807,23730.46875,32768,44370.53125,59049,77378.09375,100000,127628.1563,161051,201135.7188,248832,305175.7813,371293,448403.3438,537824,640973.4063,759375,894660.9688,1048576,1222981.031,1419857,1641308.594,1889568,2166998.656,2476099,2819506.219,3200000]);

 for i=iStart:iEnd
     t=i-single(0.5);
     A=[single(1) single(0) single(0) single(0) single(0) single(0);
        single(0) single(1) single(0) single(0) single(0) single(0);
        single(0) single(0) single(2) single(0) single(0) single(0);
        single(1) A42(i) A43(i) A44(i) A45(i) A46(i);
        single(0) single(1) A53(i) A54(i) A55(i) A56(i);
        single(0) single(0) single(2) A64(i) A65(i) A66(i)];
%     if Vterminate(i,:)==0
%         af=single(0);
%     end

% After Target Vehicle decelerates to stop,its acceleration will be zero.In order to avoid acceleration jump,target vehicle acceleration use interpolation according to its speed.
     afCoef=single(intrepolate(single(1),single(0),single(4),single(1),Vterminate(i,:)));
     af=afCoef*afRaw;
     if v0<=0
         a0=single(0);
     end
     B=[single(0) v0 a0 Dterminate(i,:) Vterminate(i,:) af];
     b=B';
     C=A\b;
     C0(i)=C(1);
     C1(i)=C(2);
     C2(i)=C(3);
     C3(i)=C(4);
     C4(i)=C(5);
     C5(i)=C(6); 

     a=single(zeros(20,40));
     adet=single(zeros(20,40));
     counterSign=single(0);
     accelSignCur=single(1);
     accelSignK1=accelSignCur;
     negAccelFadeK1=false;
     negAccelJump=false;
     velSubjTerIsTargetVel=true;
     
     jStart=single(1);
     jEnd=single(2)*t;
     for j=jStart:jEnd
            if mod(j,2)==0
                distDesPlanExpand(j)=(distDesPlan(j*single(0.5))+distDesPlan(j*single(0.5)+single(1)))*single(0.5);
                vTerminateExpand(j)=(Vterminate(j*single(0.5))+Vterminate(j*single(0.5)+single(1)))*single(0.5);
            else
                distDesPlanExpand(j)=distDesPlan((j+single(1))*single(0.5));
                vTerminateExpand(j)=Vterminate((j+single(1))*single(0.5));
            end
            if j<=jTargStop
               s(i,j)= R+vf*tBack1(j)+single(0.5)*afRaw*tBack1(j)*tBack1(j)-(C0(i) + C1(i)*tBack1(j)+ C2(i)*tBack2(j)+C3(i)*tBack3(j)+ C4(i)*tBack4(j)+ C5(i)*tBack5(j));
               v(i,j)= vf+afRaw*tBack1(j)-(C1(i) + single(2)*C2(i)*tBack1(j)+single(3)*C3(i)*tBack2(j)+single(4)*C4(i)*tBack3(j)+single(5)*C5(i)*tBack4(j));
            else
               s(i,j)= R+distTargPlan-(C0(i) + C1(i)*tBack1(j)+ C2(i)*tBack2(j) +C3(i)*tBack3(j)+ C4(i)*tBack4(j)+ C5(i)*tBack5(j));
               v(i,j)= -(C1(i) + single(2)*C2(i)*tBack1(j)+single(3)*C3(i)*tBack2(j)+single(4)*C4(i)*tBack3(j)+single(5)*C5(i)*tBack4(j));
            end
            
            velSubjPre(i,j)=C1(i) + single(2)*C2(i)*tBack1(j)+single(3)*C3(i)*tBack2(j) +single(4)*C4(i)*tBack3(j)+single(5)*C5(i)*tBack4(j);         
            a(i,j)= single(2)*C2(i) +single(6)*C3(i)*tBack1(j) +single(12)*C4(i)*tBack2(j)+single(20)*C5(i)*tBack3(j);

%% if acceleration sign translates more than twice time,J will be enlaged
            if a(i,j)<-0.1
                accelSignCur=single(-1);
            else 
                if a(i,j)>0.1
                  accelSignCur=single(1); 
                else
                  accelSignCur=accelSignK1; 
                end 
            end
            if j>=2
                if accelSignCur~=accelSignK1
                    counterSign=counterSign+single(1);
                end
            end
            accelSignK1=accelSignCur;
 %% if deceleration first gets big then gets small,and last gets 0,J will be enlaged
           if a(i,j)<-0.1
              negAccelJumpDetect=true;
           else
              negAccelJumpDetect=false;
           end
           if (j>=2)&&(negAccelJumpDetect==true)
               if (a(i,j)-a(i,j-1))>=0
                   negAccelFade=true;
                   negAccelDeep=false; 
               else
                   negAccelDeep=true;
                   negAccelFade=false;
               end
           else
               negAccelFade=false; 
               negAccelDeep=false; 
           end
           if negAccelDeep&&negAccelFadeK1
               negAccelJump=true;
           else
               negAccelJump=false;
           end
           negAccelFadeK1=negAccelFade;
 %%               
            adet(i,j)=single(6)*C3(i) +single(24)*C4(i)*tBack1(j)+single(60)*C5(i)*tBack2(j);
            velSubjNegTolerance=single(-0.3);
            
% In generally,when deceleration distance is very short,planned subjective velocity may be negtive.  For target vehicle idles,subjective vehicle override toward to target vehicle,avoiding 
% optimal solution is filted,toleranced negtive subjective velocity should be enlarged;
            if (ACCModeSts(1)==3&&ACCModeSts(2)==5)||(tOverride2Active>0.001)  
                tOverride2Active=tOverride2Active+tCycle;
            end
            if tOverride2Active>=10||ACCModeSts(1)~=3
                tOverride2Active=single(0);
            end
            if v0<8.3&&i<6&&vf>0.5&&tOverride2Active>0.001
                velSubjNegTolerance=velSubjNegTolerance+velSubjNegToleranceAdd;
            end
            if (velSubjPre(i,j)<velSubjNegTolerance)||(i==1)
               J(i,:)=single(-1);break;
            else
               accelSubjPlanTemp(i,j)=a(i,j);
               dtAccelSubjPlanTemp(i,j)=adet(i,j);
               asum(i,:)=asum(i,:)+a(i,j)^2;
               adetsum(i,:)=adetsum(i,:)+adet(i,j)^2;
               dsum(i,:)=dsum(i,:)+(s(i,j)-distDesPlanExpand(j))^2;
               vsum(i,:)=vsum(i,:)+(velSubjPre(i,j)-vTerminateExpand(j))^2;
               JadtA(i,:)=Wa*asum(i,:) +Wadet*adetsum(i,:);
               JadtADist(i,:)=Wa*asum(i,:) +Wadet*adetsum(i,:)+Wd*dsum(i,:);
            end    
     end
     if J(i,:)==-1
   
     else
        J(i,:)=Wa*asum(i,:) +Wadet*adetsum(i,:)+Wd*dsum(i,:)+Wv*vsum(i,:); 
        diffDistRelCurAbs=abs(distDesCur-R);
        diffVelRelCurAbs=abs(velTargRel);
        if (IDP0(1)==IDP0(2))
           diffAccelPlanK1Abs=abs(a(i,1)-accelSubjPlanK1);
           diffAccelPlanCurAbs=abs(a(i,1)-a0); 
        else
            diffAccelPlanK1Abs=single(0);
            diffAccelPlanCurAbs=single(0);
        end
        
        
        % stable follow 
        if (v0>3)&&(diffDistRelCurAbs<5.5)&&(diffVelRelCurAbs<2.2)
            coefJEnlarge(i)=intrepolate(single(0),single(1),single(1),single(3),diffAccelPlanK1Abs);
            coefJEnlargeTemp=intrepolate(single(0),single(1),single(1),single(3),diffAccelPlanCurAbs);
            coefJEnlarge(i)=coefJEnlarge(i)*coefJEnlargeTemp;
            coefJEnlargeNumSmall=intrepolate(single(2),single(2),single(4),single(1),i);
            coefJEnlarge(i)=coefJEnlarge(i)*coefJEnlargeNumSmall;
            J(i,:)=J(i,:)*coefJEnlarge(i);
        end
        
        % start up
        if (v0<3)&&(velTargRel>1.5)&&(a(i,1)>0.2)&&(IDP0(1)==IDP0(2))
            accelSubjPlanMax=valueMax(a(i,:),i);
            coefJEnlargeDriveOff=intrepolate(single(1.4),single(1),single(1.8),single(2),accelSubjPlanMax);
            J(i,:)=J(i,:)*coefJEnlargeDriveOff;
        end
        
        % when subjective vehicle decelerates toward to target,but situation is not dangerous,smaller i maybe selected,causing acceleration jump.In order to avoid this happen,larger decelerations i should be enlarged.
        if (ttc>3)&&(v0>3)&&(a(i,1)<-0.2)&&(IDP0(1)==IDP0(2))&&(velTargRel<-1)&&(i<=4)
            ttcEmergencyBrakThres=ttc-single(0.45);
            distBrakThresMin=intrepolate(single(-3),single(8),single(0),single(1),velTargRel);
            distBrakMax=max(distBrakThresMin,distTargRel-single(0.5)*distDesPlan(i));
            accelAverageCalc=velTargRel^2/(single(2)*distBrakMax)-single(0.5);
            accelNegSum=single(0);
            for mm=1:2*(i-0.5)
                if a(i,mm)<0
                    accelNegSum=accelNegSum+a(i,mm);
                else
                    break;
                end
            end
            accelNegAveragePlan=accelNegSum/max(single(1),(mm-single(1)));
            if t<ttcEmergencyBrakThres
                diffAccelAverage2NegAveragePlan=accelNegAveragePlan-accelAverageCalc;
            else
                diffAccelAverage2NegAveragePlan=single(0);
            end
            coefJEnlargeDecStrong=intrepolate(single(-2),single(3),single(0),single(1),diffAccelAverage2NegAveragePlan);
            J(i,:)=J(i,:)*coefJEnlargeDecStrong;
         end
     end
     
%      if counterSign>=2||negAccelJump
%          J(i,:)=single(2)*J(i,:); 
%      else
%          if velSubjTerIsTargetVel==false
%             J(i,:)=single(1)*J(i,:); 
%          end
%      end
 end
 JminIni=single(2);
 for m=2:20
     if J(m,:)==-1
         
     else
       JminIni=single(m);break;  
     end
 end
 if JminIni==20&&J(JminIni,:)==-1
     velAllIsNeg=true;
 end
 Jmin=J(JminIni,:);
 num=single(JminIni);
 numRaw=single(JminIni);
 for i=3:20
     if (J(i,:)<Jmin)&&(J(i,:)>0)
         Jmin=J(i,:);
         num=single(i);
         numRaw=single(i);
     end      
 end
 deltaJmin=abs((Jmin-J(numK1,:))/Jmin);
 if (IDP0(1)==IDP0(2))
     if deltaJmin>P_LongCtrl_FollowRateJDirStep
         
     else
         if deltaJmin>P_LongCtrl_FollowRateJConditionStep
             
          %   when subjective vehicle decelerates,if current calculated deceleration is larger 0.5 m/s^2(absolute value)than last deceleration.We can infer wether last deceleration is smaller by check planed distance.
             if (num~=numK1)&&((accelSubjPlanTemp(num,1)+0.5)<accelSubjPlanK1)&&(accelSubjPlanTemp(num,1)<-0.2)
                 distRelPlanMin= valueMin(s(numK1,:),numK1);
                 if (distRelPlanMin>5)
                     for jj=1:(2*(numK1-0.5))
                         distDesThresAccelFadeOut=intrepolate(single(10),single(0.7),single(30),single(0.6),distDesPlan(num));
                         if s(numK1,jj)<distDesThresAccelFadeOut*distDesPlanExpand(jj)
                            distRelPlanReasonable=false;break;
                         end
                     end
                     if distRelPlanReasonable==false

                     else
                        num=numK1; 
                     end
                 end
             end
             
           %  when subjective vehicle decelerates,if current calculated deceleration is smaller 0.5 m/s^2(absolute value)than last deceleration.We can infer wether last deceleration is smaller by check planed velsubj.
             if (num~=numK1)&&((accelSubjPlanTemp(num,1)>accelSubjPlanK1+0.5))&&(accelSubjPlanTemp(num,1)<-0.2)&&(velTargRel<-1)
                 velRelPlanMax= valueMax(v(num,:),num);
                 velRelPlanMaxK1= valueMax(v(numK1,:),numK1);
                 if velRelPlanMaxK1<velRelPlanMax*single(0.8)
                     num=numK1;
                 end
             end
           %  when subjective vehicle accelerates, if current calculated acceleration is smaller 0.5 m/s^2(absolute value)than last deceleration.We can infer wether last deceleration is larger by check planed velsubj.
             if (num~=numK1)&&(accelSubjPlanTemp(num,1)+0.5<accelSubjPlanK1)&&(accelSubjPlanTemp(num,1)>0.2)&&(v0<3)
                 velRelPlanMin=valueMin(v(numK1,:),numK1);
                 velRelOverShotStartUp=intrepolate(single(0),single(-2.5),single(3),single(-0.5),v0);
                 if velRelPlanMin>-0.5
                     num=numK1;
                 end
             end
           %  when subjective vehicle accelerates, if current calculated acceleration is larger 0.5 m/s^2(absolute value)than last deceleration.We can infer wether last deceleration is smaller by check planed distance.
             if (num~=numK1)&&((accelSubjPlanTemp(num,1)>accelSubjPlanK1+0.5))&&(accelSubjPlanTemp(num,1)>0.2)&&(v0<3)
                 for jj=1:(2*(numK1-0.5))
                     if s(numK1,jj)>(distDesPlanExpand(jj)+single(4))
                        distRelPlanStartReasonable=false;break;
                     end
                  end
                  if distRelPlanStartReasonable==false

                 else
                    num=numK1; 
                 end
             end
          else
              num=numK1; 
          end  
     end
 end
 if num==numK1&&num~=numRaw&&vf<P_LongCtrl_FollowVelTargetAbsSmoothNum
     if num>numRaw
        cntSmallNumRawArb=cntSmallNumRawArb+single(1);
        cntBigNumRawArb=single(0);
     else
        cntBigNumRawArb=cntBigNumRawArb+single(1);
        cntSmallNumRawArb=single(0);
     end
     if cntSmallNumRawArb>=3
         for numSmall=numRaw:(num-single(1))
             if J(numSmall,:)~=-1
                 JDiffNumSmall2Num=J(numSmall,:)-J(num,:);
                 if JDiffNumSmall2Num<=0
                    smallNumArbFail=false;
                 else
                     ratio=JDiffNumSmall2Num/J(num,:);
                    if ratio<0.1
                        smallNumArbFail=false;
                    else
                        smallNumArbFail=true;
                        break;
                    end
                 end
             end
         end
         if smallNumArbFail==false
             num=num-single(1);
         end
         cntSmallNumRawArb=single(0);
     end
     if cntBigNumRawArb>=3
         for numBig=(num+single(1)):numRaw
             if J(numBig,:)~=-1
                 JDiffNum2NumBig=J(numBig,:)-J(num,:);
                 if JDiffNum2NumBig<=0
                    BigNumArbFail=false;
                 else
                     ratio=JDiffNum2NumBig/J(num,:);
                    if ratio<0.1
                        BigNumArbFail=false;
                    else
                        BigNumArbFail=true;
                        break;
                    end
                 end
             end
         end
         if BigNumArbFail==false
             num=num+single(1);
         end
         cntBigNumRawArb=single(0);
     end
 else
    cntBigNumRawArb=single(0);
    cntSmallNumRawArb=single(0);
 end
 distRelPlan=s;
 velRelPlan=v;
 DesVelSubjPre=velSubjPre(num,:);
 DesVelSubj=single(DesVelSubjPre);
 if IDP0==uint8(0)
     distRelPlanMin= single(255);
     accelSubjpre=repmat(single(16),1,40);
     distRelDesDistRelPlanNumMin=single(255);
     distRelPlanOpt=repmat(single(255),1,40);
     velRelPlanOpt=repmat(single(255),1,40);
     DesVelSubj=repmat(single(255),1,40);
 else
     distRelPlanMin= valueMin(s(num,:),num);
     accelSubjpre=accelSubjPlanTemp(num,:);
     distRelPlanNumMin=NumMin(s(num,:),num);
     distRelDesDistRelPlanNumMin=distDesPlan(distRelPlanNumMin);
     distRelPlanOpt=s(num,:);
     velRelPlanOpt=v(num,:);
     DesVelSubjPre=velSubjPre(num,:);
     DesVelSubj=single(DesVelSubjPre);
 end
 accelSubjPlan=single(accelSubjpre);
function result=intrepolate(x1,y1,x2,y2,x)
if x<x1
    result=single(y1);
else
    if x>x2
        result=single(y2);
    else
        result=single(y1+(y2-y1)/(x2-x1)*(x-x1));
    end
end
function resultMin=valueMin(PlanOptTemp,numOpt)
resultMin=PlanOptTemp(1);
iiEnd=single(2)*(numOpt-single(0.5));
for ii=single(2):iiEnd
    if PlanOptTemp(ii)<resultMin
       resultMin=PlanOptTemp(ii);
    end
end
function PointMin=NumMin(PlanOptTemp1,numOpt1)
resultMin1=PlanOptTemp1(1);
PointMin=single(1);
iiEnd=single(2)*(numOpt1-single(0.5));
for ii=single(2):iiEnd
    if PlanOptTemp1(ii)<resultMin1
       resultMin1=PlanOptTemp1(ii);
       PointMin=single(ceil(ii/single(2)));
    end
end
function resultMax=valueMax(PlanOptTemp2,numOpt2)
resultMax=PlanOptTemp2(1);
iiEnd=single(2)*(numOpt2-single(0.5));
for ii=single(2):iiEnd
    if PlanOptTemp2(ii)>resultMax
       resultMax=PlanOptTemp2(ii);
    end
end
